simulink model "robot_dinamica"  (R2021a)
settings: Solver=ode45  StartTime=0.0  StopTime=4  MaxStep=1e-3  RelTol=1e-3
undefined symbols (not defined in the file or in its folder): CinematicaInversa, Kd1, Kd2, Kd3, Ki1, Ki2, Ki3, Kp1, Kp2, Kp3
settings Model: Creator=Pablo Carmona  LastModifiedBy=Pablo Carmona

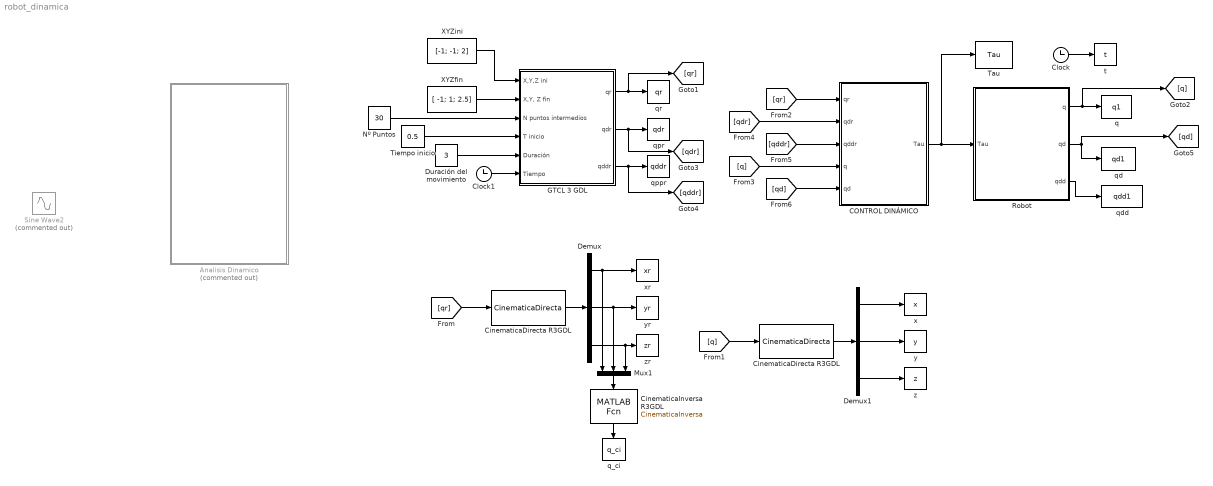
== system robot_dinamica ==
  Analisis Dinamico : Subsystem  Commented=on
  CONTROL DINÁMICO : Subsystem
  CinematicaDirecta R3GDL : MATLABFcn  MATLABFcn=CinematicaDirecta  OutputDimensions=3
  "CinematicaDirecta R3GDL " : MATLABFcn  MATLABFcn=CinematicaDirecta  OutputDimensions=3
  CinematicaInversa R3GDL : MATLABFcn  MATLABFcn=CinematicaInversa  OutputDimensions=3
  Clock : Clock
  Clock1 : Clock
  Demux : Demux  Outputs=3
  Demux1 : Demux  Outputs=3
  Duración del movimiento : Constant  Value=3
  GTCL 3 GDL : Subsystem
  Mux1 : Mux  Inputs=3
  Nº Puntos : Constant  Value=30
  Robot : Subsystem
      mask Display: image('esquema3gdl_limpio.jpg'); % Use "Edit Image" on toolstrip to change.
  Sine Wave2 : Sin  Commented=on  Frequency=10  SampleTime=0
  "Tau " : ToWorkspace  VariableName=Tau  SampleTime=-1
  Tiempo inicio : Constant  Value=0.5
  XYZfin : Constant  Value=[ -1; 1; 2.5]
  XYZini : Constant  Value=[-1; -1; 2]
  q : ToWorkspace  VariableName=q1  SampleTime=-1
  q_ci : ToWorkspace  VariableName=q_ci  SaveFormat=Structure With Time  SampleTime=-1
  qd : ToWorkspace  VariableName=qd1  SampleTime=-1
  qdd : ToWorkspace  VariableName=qdd1  SampleTime=-1
  qppr : ToWorkspace  VariableName=qddr  SaveFormat=Structure With Time  SampleTime=-1
  qpr : ToWorkspace  VariableName=qdr  SaveFormat=Structure With Time  SampleTime=-1
  qr : ToWorkspace  VariableName=qr  SaveFormat=Structure With Time  SampleTime=-1
  t : ToWorkspace  VariableName=t  SampleTime=-1
  x : ToWorkspace  VariableName=x  SampleTime=-1
  xr : ToWorkspace  VariableName=xr  SampleTime=-1
  y : ToWorkspace  VariableName=y  SampleTime=-1
  yr : ToWorkspace  VariableName=yr  SampleTime=-1
  z : ToWorkspace  VariableName=z  SampleTime=-1
  zr : ToWorkspace  VariableName=zr  SampleTime=-1
  wires:
  Demux/1 -> xr/1, Mux1/1
  CinematicaDirecta R3GDL/1 -> Demux/1
  Demux/3 -> Mux1/3, zr/1
  [qr] -> CinematicaDirecta R3GDL/1
  Tiempo inicio/1 -> GTCL 3 GDL/4(T inicio)
  Nº Puntos/1 -> GTCL 3 GDL/3(N puntos intermedios)
  GTCL 3 GDL/2(qdr) -> qpr/1, [qdr]
  Clock1/1 -> GTCL 3 GDL/6(Tiempo)
  XYZini/1 -> GTCL 3 GDL/1(X,Y,Z ini)
  Duración del movimiento/1 -> GTCL 3 GDL/5(Duración)
  GTCL 3 GDL/1(qr) -> qr/1, [qr]
  XYZfin/1 -> GTCL 3 GDL/2("X,Y, Z fin")
  Mux1/1 -> CinematicaInversa R3GDL/1
  Demux/2 -> yr/1, Mux1/2
  CinematicaInversa R3GDL/1 -> q_ci/1
  Demux1/3 -> z/1
  [qd] -> CONTROL DINÁMICO/5(qd)
  [q] -> CONTROL DINÁMICO/4(q)
  Demux1/1 -> x/1
  [qdr] -> CONTROL DINÁMICO/2(qdr)
  [q] -> "CinematicaDirecta R3GDL "/1
  "CinematicaDirecta R3GDL "/1 -> Demux1/1
  CONTROL DINÁMICO/1(Tau) -> "Tau "/1, Robot/1(Tau)
  [qddr] -> CONTROL DINÁMICO/3(qddr)
  Demux1/2 -> y/1
  Robot/2(qd) -> qd/1, [qd]
  Clock/1 -> t/1
  Robot/3(qdd) -> qdd/1
  Robot/1(q) -> [q], q/1
  [qr] -> CONTROL DINÁMICO/1(qr)
  GTCL 3 GDL/3(qddr) -> [qddr], qppr/1

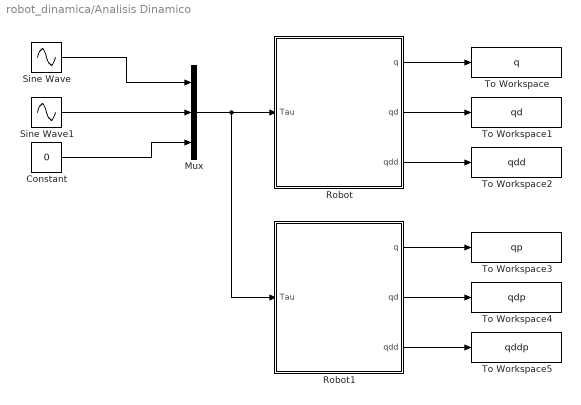
== system robot_dinamica/Analisis Dinamico ==
  Constant : Constant  Value=0
  Mux : Mux  Inputs=3
  Robot : Subsystem
      mask Display: image('captura_esquema_3GDL_cleanup.png'); % Use "Edit Image" on toolstrip to change.
  Robot1 : Subsystem
      mask Display: image('esquema3gdl_limpio.jpg'); % Use "Edit Image" on toolstrip to change.
  Sine Wave : Sin  Amplitude=0.5  SampleTime=0
  Sine Wave1 : Sin  Amplitude=0.5  SampleTime=0
  To Workspace : ToWorkspace  VariableName=q  SaveFormat=Structure With Time  SampleTime=-1
  To Workspace1 : ToWorkspace  VariableName=qd  SaveFormat=Structure With Time  SampleTime=-1
  To Workspace2 : ToWorkspace  VariableName=qdd  SaveFormat=Structure With Time  SampleTime=-1
  To Workspace3 : ToWorkspace  VariableName=qp  SaveFormat=Structure With Time  SampleTime=-1
  To Workspace4 : ToWorkspace  VariableName=qdp  SaveFormat=Structure With Time  SampleTime=-1
  To Workspace5 : ToWorkspace  VariableName=qddp  SaveFormat=Structure With Time  SampleTime=-1
  wires:
  Mux/1 -> Robot1/1(Tau), Robot/1(Tau)
  Robot1/3(qdd) -> To Workspace5/1
  Robot/2(qd) -> To Workspace1/1
  Robot/1(q) -> To Workspace/1
  Sine Wave1/1 -> Mux/2
  Robot1/2(qd) -> To Workspace4/1
  Robot/3(qdd) -> To Workspace2/1
  Constant/1 -> Mux/3
  Robot1/1(q) -> To Workspace3/1
  Sine Wave/1 -> Mux/1

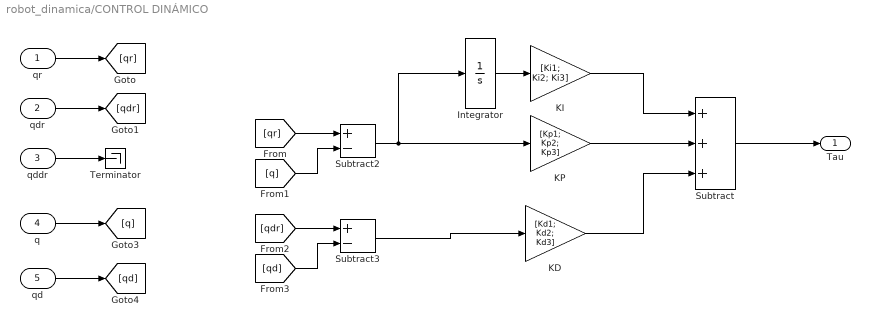
== system robot_dinamica/CONTROL DINÁMICO ==
  qr : Inport
  qdr : Inport  Port=2
  qddr : Inport  Port=3
  q : Inport  Port=4
  qd : Inport  Port=5
  Integrator : Integrator
  KD : Gain  Gain=[Kd1; Kd2; Kd3]
  KI : Gain  Gain=[Ki1; Ki2; Ki3]
  KP : Gain  Gain=[Kp1; Kp2; Kp3]
  Subtract : Sum  Inputs=+++
  Subtract2 : Sum  Inputs=+-
  Subtract3 : Sum  Inputs=+-
  Terminator : Terminator
  Tau : Outport
  wires:
  Subtract/1 -> Tau/1
  Subtract2/1 -> Integrator/1, KP/1
  Subtract3/1 -> KD/1
  qr/1 -> [qr]
  qdr/1 -> [qdr]
  qddr/1 -> Terminator/1
  q/1 -> [q]
  qd/1 -> [qd]
  [qr] -> Subtract2/1
  [q] -> Subtract2/2
  [qdr] -> Subtract3/1
  [qd] -> Subtract3/2
  KI/1 -> Subtract/1
  KP/1 -> Subtract/2
  KD/1 -> Subtract/3
  Integrator/1 -> KI/1

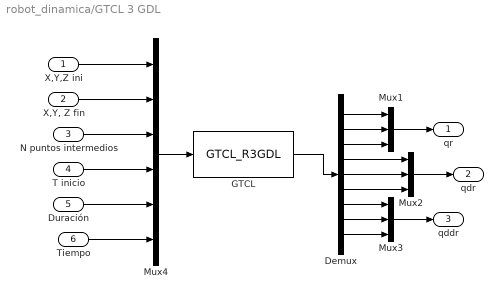
== system robot_dinamica/GTCL 3 GDL ==
  X,Y,Z ini : Inport
  "X,Y, Z fin" : Inport  Port=2
  N puntos intermedios : Inport  Port=3
  T inicio : Inport  Port=4
  Duración : Inport  Port=5
  Tiempo : Inport  Port=6
  Demux : Demux  Outputs=9
  GTCL : MATLABFcn  MATLABFcn=GTCL_R3GDL  OutputDimensions=9
  Mux1 : Mux  Inputs=3
  Mux2 : Mux  Inputs=3
  Mux3 : Mux  Inputs=3
  Mux4 : Mux  Inputs=6
  qr : Outport
  qdr : Outport  Port=2
  qddr : Outport  Port=3
  wires:
  Mux1/1 -> qr/1
  Mux4/1 -> GTCL/1
  X,Y,Z ini/1 -> Mux4/1
  "X,Y, Z fin"/1 -> Mux4/2
  N puntos intermedios/1 -> Mux4/3
  T inicio/1 -> Mux4/4
  Duración/1 -> Mux4/5
  Tiempo/1 -> Mux4/6
  GTCL/1 -> Demux/1
  Demux/1 -> Mux1/1
  Demux/2 -> Mux1/2
  Demux/3 -> Mux1/3
  Mux2/1 -> qdr/1
  Demux/4 -> Mux2/1
  Demux/5 -> Mux2/2
  Demux/6 -> Mux2/3
  Mux3/1 -> qddr/1
  Demux/7 -> Mux3/1
  Demux/8 -> Mux3/2
  Demux/9 -> Mux3/3

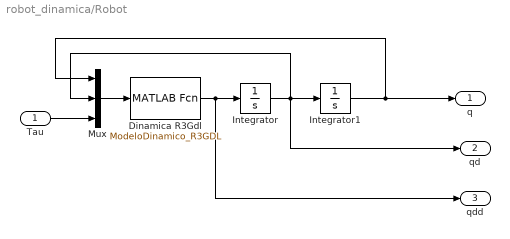
== system robot_dinamica/Robot ==
  Tau : Inport
  Dinamica R3Gdl : MATLABFcn  MATLABFcn=ModeloDinamico_R3GDL  OutputDimensions=3
  Integrator : Integrator  InitialCondition=[0;0;0];
  Integrator1 : Integrator  InitialCondition=CinematicaInversa([0.5; 0; 1])
  Mux : Mux  Inputs=3
  q : Outport
  qd : Outport  Port=2
  qdd : Outport  Port=3
  wires:
  Mux/1 -> Dinamica R3Gdl/1
  Dinamica R3Gdl/1 -> Integrator/1, qdd/1
  Integrator/1 -> Integrator1/1, qd/1, Mux/2
  Integrator1/1 -> q/1, Mux/1
  Tau/1 -> Mux/3

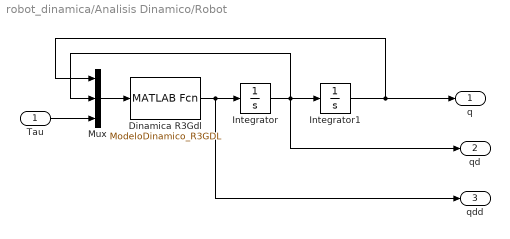
== system robot_dinamica/Analisis Dinamico/Robot ==
  Tau : Inport
  Dinamica R3Gdl : MATLABFcn  MATLABFcn=ModeloDinamico_R3GDL  OutputDimensions=3
  Integrator : Integrator  InitialCondition=[0;0;0];
  Integrator1 : Integrator  InitialCondition=[0,0,0]
  Mux : Mux  Inputs=3
  q : Outport
  qd : Outport  Port=2
  qdd : Outport  Port=3
  wires:
  Mux/1 -> Dinamica R3Gdl/1
  Dinamica R3Gdl/1 -> Integrator/1, qdd/1
  Integrator/1 -> Integrator1/1, qd/1, Mux/2
  Integrator1/1 -> q/1, Mux/1
  Tau/1 -> Mux/3

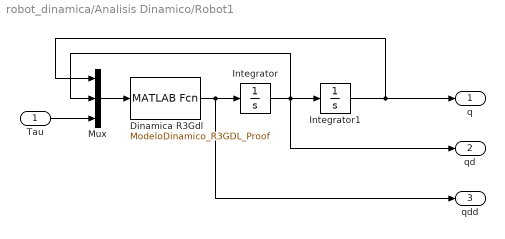
== system robot_dinamica/Analisis Dinamico/Robot1 ==
  Tau : Inport
  Dinamica R3Gdl : MATLABFcn  MATLABFcn=ModeloDinamico_R3GDL_Proof  OutputDimensions=3
  Integrator : Integrator  InitialCondition=[0;0;0];
  Integrator1 : Integrator  InitialCondition=[0,0,0]
  Mux : Mux  Inputs=3
  q : Outport
  qd : Outport  Port=2
  qdd : Outport  Port=3
  wires:
  Mux/1 -> Dinamica R3Gdl/1
  Dinamica R3Gdl/1 -> Integrator/1, qdd/1
  Integrator/1 -> Integrator1/1, qd/1, Mux/2
  Integrator1/1 -> q/1, Mux/1
  Tau/1 -> Mux/3
